simulink model "foucaultSubs_Shelby"  (R2018b)
settings: Solver=ode23t  StartTime=0.0  StopTime=3600  FixedStep=.1  RelTol=1e-5  EnableMultiTasking=on
PreLoadFcn:
  | g = 9.83;          % acceleration of gravity (m/sec^2)
  | L = 67;            % pendulum length (m)
  | initial_x = L/100; % initial x coordinate (m)
  | initial_y = 0;     % initial y coordinate (m)
  | initial_xdot = 0;  % initial x velocity (m/sec)
  | initial_ydot = 0;  % initial y velocity (m/sec)
  | Omega=2*pi/86400;  % Earth's angular velocity of rotation about its axis (rad/sec)
  | lambda=49/180*pi;  % latitude in (rad)
CloseFcn:
  | close(findobj('Tag','CloseMe'));
settings Model: Creator=The MathWorks Inc.  LastModifiedBy=shelbyjohnson
settings DataIOCC: SaveFormat=StructureWithTime  SaveOutput=off  SaveTime=off  SignalLoggingName=sldemo_foucault_output
settings OptimizationCC: ExpressionDepthLimit=2147483647  InitFltsAndDblsToZero=on  LifeSpan=inf
settings DebuggingCC: SaveWithParameterizedLinksMsg=none  UnderspecifiedInitializationDetection=Classic  MergeDetectMultiDrivingBlocksExec=none  SignalResolutionControl=TryResolveAllWithWarning  ParameterPrecisionLossMsg=none  FcnCallInpInsideContextMsg=warning  AllowSymbolicDim=off  StateNameClashWarn=warning  LibraryContextMissingDiagnostic=none  SFUnexpectedBacktrackingDiag=warning  SFNoUnconditionalDefaultTransitionDiag=warning  SFExecutionAtInitializationDiag=none
settings HardwareCC: ProdBitPerPointer=32  ProdBitPerSizeT=32  ProdBitPerPtrDiffT=32  ProdLargestAtomicFloat=None  ProdIntDivRoundTo=Undefined  ProdEndianess=Unspecified  ProdWordSize=32  ProdHWDeviceType=32-bit Generic
settings ModelReferenceCC: PropagateSignalLabelsOutOfModel=off
settings SFSimCC: SimUseLocalCustomCode=off
settings RTWCC: RTWUseLocalCustomCode=off
settings CodeAppCC: StateflowObjectComments=on
settings GRTTargetCC: TargetFcnLib=ansi_tfl_tmw.mat  TargetLangStandard=C89/C90 (ANSI)  GeneratePreprocessorConditionals=Disable all  CombineOutputUpdateFcns=off  GRTInterface=on
settings ConfigComp: CovMetricSettings=dw  CovHtmlReporting=on  CovSaveCumulativeToWorkspaceVar=on  CovSaveSingleToWorkspaceVar=on  CovExternalEMLEnable=off  CovSFcnEnable=off

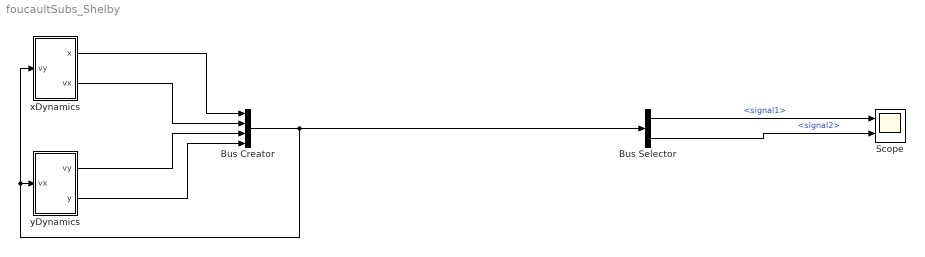
== system foucaultSubs_Shelby ==
  Bus Creator : BusCreator  Inputs=4
  Bus Selector : BusSelector  OutputSignals=signal1,signal2
  Scope : Scope  NumInputPorts=2
  xDynamics : Subsystem
  yDynamics : Subsystem
  wires:
  xDynamics/1(x) -> Bus Creator/1
  xDynamics/2(vx) -> Bus Creator/2
  yDynamics/1(vy) -> Bus Creator/3
  yDynamics/2(y) -> Bus Creator/4
  Bus Creator/1 -> yDynamics/1(vx), xDynamics/1(vy), Bus Selector/1
  Bus Selector/1 -> Scope/1  "<signal1>"
  Bus Selector/2 -> Scope/2  "<signal2>"

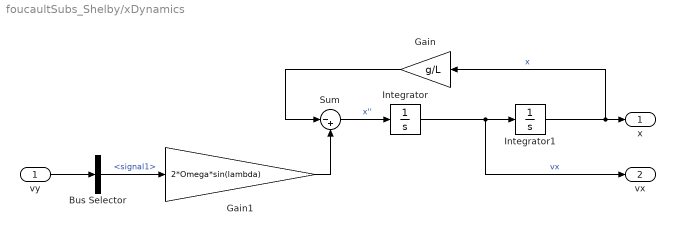
== system foucaultSubs_Shelby/xDynamics ==
  vy : Inport
  Bus Selector : BusSelector  OutputSignals=signal1
  Gain : Gain  Gain=g/L
  Gain1 : Gain  Gain=2*Omega*sin(lambda)
  Integrator : Integrator  InitialCondition=initial_xdot
  Integrator1 : Integrator  InitialCondition=initial_x
  Sum : Sum  Inputs=|-+
  x : Outport
  vx : Outport  Port=2
  wires:
  Integrator/1 -> Integrator1/1, vx/1  "vx"
  Integrator1/1 -> Gain/1, x/1  "x"
  Sum/1 -> Integrator/1  "x''"
  Gain/1 -> Sum/1
  Gain1/1 -> Sum/2
  vy/1 -> Bus Selector/1
  Bus Selector/1 -> Gain1/1  "<signal1>"

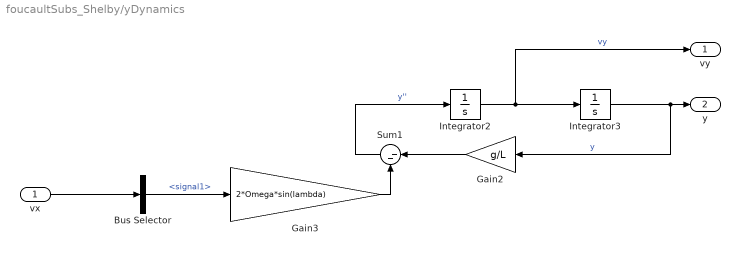
== system foucaultSubs_Shelby/yDynamics ==
  vx : Inport
  Bus Selector : BusSelector  OutputSignals=signal1
  Gain2 : Gain  Gain=g/L
  Gain3 : Gain  Gain=2*Omega*sin(lambda)
  Integrator2 : Integrator  InitialCondition=initial_ydot
  Integrator3 : Integrator  InitialCondition=initial_y
  Sum1 : Sum  Inputs=|--
  vy : Outport
  y : Outport  Port=2
  wires:
  Integrator2/1 -> Integrator3/1, vy/1  "vy"
  Gain2/1 -> Sum1/1
  Gain3/1 -> Sum1/2
  Sum1/1 -> Integrator2/1  "y''"
  Integrator3/1 -> Gain2/1, y/1  "y"
  vx/1 -> Bus Selector/1
  Bus Selector/1 -> Gain3/1  "<signal1>"
